simulink model "New_2"  (R2020a)
settings: Solver=VariableStepAuto  StartTime=0.0  StopTime=0.3  MaxStep=1e-5  RelTol=1e-3  EnableMultiTasking=on
libraries: simulink x1
settings Model: SimulationMode=accelerator  Creator=OXAALJ  LastModifiedBy=galarm2
settings SolverCC: MaxOrder=2  MaxConsecutiveZCs=10  MaxConsecutiveMinStep=10  ZeroCrossControl=DisableAll
settings DataIOCC: LimitDataPoints=on  SaveFormat=Array  DSMLogging=off  ReturnWorkspaceOutputs=off
settings OptimizationCC: LifeSpan=inf
settings DebuggingCC: UnderspecifiedInitializationDetection=Classic  MergeDetectMultiDrivingBlocksExec=none  SolverPrmCheckMsg=warning  MultiTaskDSMMsg=warning  MultiTaskCondExecSysMsg=none  StateNameClashWarn=warning  SFUnexpectedBacktrackingDiag=warning  SFNoUnconditionalDefaultTransitionDiag=warning  SFExecutionAtInitializationDiag=none  ArithmeticOperatorsInVariantConditions=warning
settings HardwareCC: ProdBitPerPointer=32  ProdBitPerSizeT=32  ProdBitPerPtrDiffT=32  ProdLargestAtomicFloat=None  ProdIntDivRoundTo=Undefined  ProdEndianess=Unspecified  ProdWordSize=32  ProdHWDeviceType=32-bit Generic
settings ModelReferenceCC: PropagateSignalLabelsOutOfModel=off
settings SFSimCC: SimUseLocalCustomCode=off  CustomCodeUndefinedFunction=UseInterfaceOnly
settings RTWCC: RTWUseLocalCustomCode=off
settings CodeAppCC: StateflowObjectComments=on
settings GRTTargetCC: TargetLangStandard=C89/C90 (ANSI)
settings ConfigComp: CovMetricSettings=dw  CovHtmlReporting=on  CovSaveCumulativeToWorkspaceVar=on  CovSaveSingleToWorkspaceVar=on  CovExternalEMLEnable=off  CovSFcnEnable=off

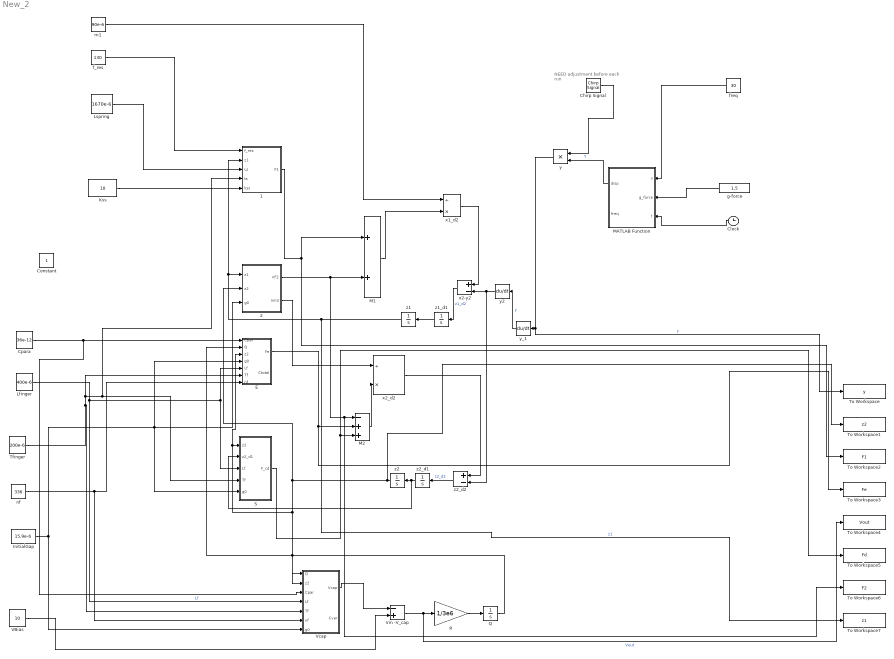
== system New_2 ==
  note: NEED
      | adjustment
      | before each
      | run
  " M1" : Sum  RndMeth=Nearest
  1 : MATLAB Function  TreatAsAtomicUnit=on
  2 : MATLAB Function  TreatAsAtomicUnit=on
  Chirp Signal : simulink/Sources/Chirp Signal  f1=30  T=0.3  f2=30
  Clock : Clock
  Cpara : Constant  Value=36e-12  VectorParams1D=off
  E : MATLAB Function  TreatAsAtomicUnit=on
  InitialGap : Constant  Value=15.9e-6
  Kss : Constant  Value=10
  Lfinger : Constant  Value=400e-6
  Lspring : Constant  Value=1670e-6
  M2 : Sum  Inputs=-++  RndMeth=Nearest
  MATLAB Function : MATLAB Function  TreatAsAtomicUnit=on
  Q : Integrator
  R : Gain  Gain=1/3e6
  S : MATLAB Function  TreatAsAtomicUnit=on
  Tfinger : Constant  Value=200e-6
  To Workspace : ToWorkspace  VariableName=y  SampleTime=-1
      settings: Save2DSignal=2-D array (concatenate along first dimension)
  To Workspace1 : ToWorkspace  VariableName=z2  SampleTime=-1
      settings: Save2DSignal=2-D array (concatenate along first dimension)
  To Workspace2 : ToWorkspace  VariableName=F1  SampleTime=-1
      settings: Save2DSignal=2-D array (concatenate along first dimension)
  To Workspace3 : ToWorkspace  VariableName=Fe  SampleTime=-1
      settings: Save2DSignal=2-D array (concatenate along first dimension)
  To Workspace4 : ToWorkspace  VariableName=Vout  SampleTime=-1
      settings: Save2DSignal=2-D array (concatenate along first dimension)
  To Workspace5 : ToWorkspace  VariableName=Fd  SampleTime=-1
      settings: Save2DSignal=2-D array (concatenate along first dimension)
  To Workspace6 : ToWorkspace  VariableName=F2  SampleTime=-1
      settings: Save2DSignal=2-D array (concatenate along first dimension)
  To Workspace7 : ToWorkspace  VariableName=z1  SampleTime=-1
      settings: Save2DSignal=2-D array (concatenate along first dimension)
  VBias : Constant  Value=10
  Vcap : MATLAB Function  TreatAsAtomicUnit=on
  Vin -V_cap : Sum  Inputs=-+  RndMeth=Nearest
  f_res : Constant  Value=130
  freq : Constant  Value=30
  g-force : Constant  Value=1.5
  m1 : Constant  Value=90e-6
  nf : Constant  Value=336
  x1_d2 : Product  Inputs=/*
  x2-y2 : Sum  Inputs=+-  RndMeth=Nearest
  x2_d2 : Product  Inputs=/*
  y : Product
  y2 : Derivative
  y_1 : Derivative
  z1 : Integrator
  z1_d1 : Integrator
  z2 : Integrator
  z2_d1 : Integrator
  z2_d2 : Sum  Inputs=+-  RndMeth=Nearest
  Constant : Constant  IOType=siggen
  wires:
  E/1(Fe) -> To Workspace3/1, M2/2
  1/1(F1) -> To Workspace2/1, " M1"/1
  S/1(F_cd) -> To Workspace5/1, M2/3
  f_res/1 -> 1/1(f_res)
  m1/1 -> x1_d2/1
  Clock/1 -> MATLAB Function/3(t)
  g-force/1 -> MATLAB Function/2(g_force)
  freq/1 -> MATLAB Function/1(f)
  MATLAB Function/1(disp) -> y/2  "Y"
  y/1 -> To Workspace/1, y_1/1  "y"
  InitialGap/1 -> E/4(g0), S/5(g0), 2/3(g0), Vcap/7(g0)
  VBias/1 -> Vin -V_cap/2
  Vin -V_cap/1 -> To Workspace4/1, R/1  "Vout"
  R/1 -> Q/1
  Q/1 -> E/2(Q), Vcap/1(Q)
  Vcap/1(Vcap) -> Vin -V_cap/1
  Lfinger/1 -> Vcap/4(Lf), E/5(Lf), S/3(Lf)  "Lf"
  Cpara/1 -> Vcap/3(Cpar), E/1(Cpar)
  Chirp Signal/1 -> y/1
  nf/1 -> Vcap/6(nf), E/7(nf)
  Lspring/1 -> 1/3(Ls)
  Tfinger/1 -> E/6(Tf), 1/4(ts), S/4(Tf), Vcap/5(Tf)
  Kss/1 -> 1/5(kss)
  2/1(nF2) -> To Workspace6/1, M2/1, " M1"/2
  " M1"/1 -> x1_d2/2
  y_1/1 -> y2/1  "y"
  x1_d2/1 -> x2-y2/1
  y2/1 -> z2_d2/2, x2-y2/2
  x2-y2/1 -> z1_d1/1  "z1_d2"
  z1_d1/1 -> z1/1
  z1/1 -> To Workspace7/1, 1/2(z1), 2/1(z1)  "z1"
  x2_d2/1 -> z2_d2/1
  z2_d2/1 -> z2_d1/1  "z2_d2"
  z2_d1/1 -> S/2(z2_d1), z2/1
  z2/1 -> To Workspace1/1, Vcap/2(z2), S/1(z2), E/3(z2), 2/2(z2)
  2/2(nm2) -> x2_d2/1
  M2/1 -> x2_d2/2

== matlab function New_2/E ==
  data: Cpar input; Q input; Fe output; z2 input; g0 input; Ctotal output; Lf input; Tf input; nf input
function [Fe,Ctotal] = fcn(Cpar,Q,z2,g0,Lf,Tf,nf)
% This function is to calculate the Fe (electrostatic force on m2)


%%%% slanted electrodes (BASSET 2014)
a = 3.5/200;    %aspect ratio
%C = ((eps0.*nf.*Lf)./(4.*a)).*log( ((g+2.*Wf.*a).^2 - z2.^2)./ (g.^2 - z2.^2));
% Cfit = (4.58916e18)*z2^6 - (6.34823e10)*z2^5 - (8.01379e8)*z2^4 + ...
%     (1.06902e1)*z2^3 + (8.85118e-2)*z2^2 + (3.66175e-11)*z2 + 1.50912e-11; % from excel
%Ctotal = Cfit + Cpar;
%==========================================================================
% Accounting for Parylene

eps0 = 8.85e-12;                                %permitivity of free space 
er   = 3.15;                                    %relative dielectric (Parylene C)
t    = 200e-9;                                  % thickness of parylene
g_p  = g0 - 2*t;                                % Minimum air gap
Ctot = 0;                                       % this gets reassigned in the if statements
z2lin = 1.54e-5;                              % z2 value at which linear approx starts
dcdz2 = 0.0605;                                % Slope of linear approx
c0 = 1.1855e-10;                                % Capacitance value at z2lin

if g_p > abs(z2)    %separate motion
    z2 = z2 * 2;
    C_L = ((eps0.*Lf)./(2.*a)).*( log( (g_p + z2 + 2.*a.*Tf)./(g_p + z2) ) );
    C_Leff = 1./( (2./(er.*eps0.*Lf.*Tf./t)) + 1./C_L);
    
    C_R = ((eps0.*Lf)./(2.*a)).*( log( (g_p - z2 + 2.*a.*Tf)./(g_p - z2) ) );
    C_Reff = 1 ./ ( (2./(er.*eps0.*Lf.*Tf./t)) + 1./C_R);

    Ctot = (C_Leff + C_Reff).*(nf./2);    
end

if -z2lin > z2      % Impacting with Left Hand side
    Ctot = c0 + dcdz2.*(-g_p - z2); 
end 

if z2 > z2lin      % impacting with RHS
    Ctot = c0 + dcdz2.*(z2 - g_p);
end

Ctotal = Ctot + Cpar;
% z2max = 15.5e-6;     %maximum displaccement for capacitance calc
% Cmax = (4.58916e18)*z2max^6 - (6.34823e10)*z2max^5 - (8.01379e8)*z2max^4 + ...
%     (1.06902e1)*z2max^3 + (8.85118e-2)*z2max^2 + (3.66175e-11)*z2max...
%     + 1.50912e-11;      %capacitance at z2max
% C = min(Cmax,Cfit);     % Use Cmax if z2>z2max


% dC is divided by four here because nf is total electrodes, not number of
% electrode pairs
dC = ((eps0.*nf.*Lf)./(4.*a))*( ((2*z2)/(g0^2 - z2^2)) - ((2*z2)/((g0+2*Tf*a)^2 - z2^2) ));

% dC = ((eps0.*nf.*Lf)./(1*a))*( ((2*z2)/(g0^2 - z2^2)) - ((2*z2)/((g0+2*Tf*a)^2 - z2^2) ));  % Nf IS the number of electrodes

Fe = -1*((Q^2)/(2*Ctotal^2))*dC;


end

== matlab function New_2/S ==
  data: z2 input; F_cd output; z2_d1 input; Lf input; Tf input; g0 input
function F_cd  = SQFD(z2,z2_d1,Lf,Tf,g0)
% This block supports an embeddable subset of the MATLAB language.
% See the help menu for details. 


mu = 1.846e-5;      %dynamic viscosity of air

%--------------------------------------------------------------------------
%Simple, low amplitude SQFD
% cd = nf*mu*Lf*Wf^3.*(1./(g-z).^3 + 1./(g+z).^3);
% A   = 14.4e-6;      %Soft Stopper Nominal Gap (meters)
% 
t    = 200e-9;                                  % thickness of parylene
g_p  = g0 - 2*t;                                % Minimum air gap


if  abs (z2) < g_p    %the separate motion
    z2 = 2*z2;
    z2_d1 = 2*z2_d1;
end   
% 
% b_eff   =   1.3;                                      % boarder effect coefficient
% epsr    =   3.15;                                     % relative dielectric
% 
% 
% tf_r    =   Tf + b_eff * ( g_p - z2 );
% tf_l    =   Tf + b_eff * ( g_p + z2 );
% lf_r    =   Lf + b_eff * ( g_p - z2 );
% lf_l    =   Lf + b_eff * ( g_p + z2 );
% 
% cdr     =   nf * mu * lf_r * tf_r^3 * ( g_p - z2  ) ^(-3) ;
% cdl     =   nf * mu * lf_l * tf_l^3 * ( g_p + z2  ) ^(-3) ;
% 
% F_cd      =   - 1*( cdr + cdl ) * z2_d1 ; 


%-----------The classic squeeze film damping equation------------%
% 
% tp        =   200e-9;                                     % the thickness of paralyene
% Cd        =   20e-20;  
% epsr      =   3.15;                                       % relative dielectric
% 
% F_cd        =   -Cd * z2_d1* (( g_p  - z2 + 2*tp/epsr) ^(-3) + ( g_p  + z2 + 2*tp/epsr) ^(-3));

%% Andy Moy damping original
% mu    =   1.983e-5;                                   %Air viscocity dynamic (kg/m*s)
% rho   =   1.204;                                      %Air density    (kg/m3)                    
% a     =   3.5*2/200;                                  %Tilt angle difference, tan(a)- tan(b)
% 
% 
% t    = 200e-9;                                  % thickness of parylene
% g_p  = g0 - 2*t;                                % Minimum air gap
% % Left-hand side
% 
% ho_l  =  g_p + z2;                                    %Left-hand side ho
% hl_l  =  ho_l + a*Tf;                                %Left-hand side hl
% 
% C1_l  =  -ho_l*Tf/(ho_l + 2*a)* z2_d1;               %The c1 parameter, left
% C2_l  =  12*mu*a^-2/(2*ho_l + a*Tf) * z2_d1;         %The c1 parameter, left
% 
% 
% F_l   =  Lf * (Tf * C2_l - 6*mu*Tf/a/ho_l/hl_l*C1_l + 6*mu*Tf*a^-4/hl_l*z2_d1+ 12*mu*a^-3 * z2_d1 * (log(ho_l./hl_l)) ); 
% % F_l   =  Lf * (Tf * C2_l - 6*mu*Tf/a/ho_l/hl_l*C1_l + 6*mu*Tf*a^-4/hl_l*z2_d1+ 12*mu*a^-3 * z2_d1 * (log(16/22)) ); 
% % Right-hand side                   
% 
% ho_r  =  g_p - z2;                                    %Left-hand side ho
% hl_r  =  ho_r + a*Tf;                                %Left-hand side hl
% 
% C1_r  =  -ho_r*Tf/(ho_r + 2*a)* z2_d1;                 %The c1 parameter, right
% C2_r  =  12*mu*a^-2/(2*ho_r + a*Tf) * z2_d1;         %The c1 parameter, right
% 
% 
% F_r   =  Lf * (Tf * C2_r - 6*mu*Tf/a/ho_r/hl_r*C1_r + 6*mu*Tf*a^-4/hl_r*z2_d1 + 12*mu*a^-3 * z2_d1 * (log(ho_r./hl_r) )) ; 
% % F_r   =  Lf * (Tf * C2_r - 6*mu*Tf/a/ho_r/hl_r*C1_r + 6*mu*Tf*a^-4/hl_r*z2_d1 + 12*mu*a^-3 * z2_d1 * (log(16/22) )) ; 
% F_cd  =  -100000*(F_l  + F_r)*nf;


%% Andy Moy damping Tf Lf
mu    =   1.983e-5;                                   %Air viscocity dynamic (kg/m*s)
rho   =   1.204;                                      %Air density    (kg/m3)                    
a     =   3.5*2/200;                                  %Tilt angle difference, tan(a)- tan(b)


t    = 200e-9;                                  % thickness of parylene
g_p  = g0 - 2*t;                                % Minimum air gap
% Left-hand side

ho_l  =  g_p + z2;                                    %Left-hand side ho
hl_l  =  ho_l + a*Lf;                                %Left-hand side hl

C1_l  =  -ho_l*Lf/(ho_l + 2*a)* z2_d1;               %The c1 parameter, left
C2_l  =  12*mu*a^-2/(2*ho_l + a*Lf) * z2_d1;         %The c1 parameter, left


F_l   =  Tf * (Lf * C2_l - 6*mu*Lf/a/ho_l/hl_l*C1_l + 6*mu*Lf*a^-4/hl_l*z2_d1+ 12*mu*a^-3 * z2_d1 * (log(ho_l./hl_l)) )*0.336; 
% F_l   =  Lf * (Tf * C2_l - 6*mu*Tf/a/ho_l/hl_l*C1_l + 6*mu*Tf*a^-4/hl_l*z2_d1+ 12*mu*a^-3 * z2_d1 * (log(16/22)) ); 
% Right-hand side                   

ho_r  =  g_p - z2;                                    %Left-hand side ho
hl_r  =  ho_r + a*Lf;                                %Left-hand side hl

C1_r  =  -ho_r*Lf/(ho_r + 2*a)* z2_d1;                 %The c1 parameter, right
C2_r  =  12*mu*a^-2/(2*ho_r + a*Lf) * z2_d1;         %The c1 parameter, right


F_r   =  Tf * (Lf * C2_r - 6*mu*Lf/a/ho_r/hl_r*C1_r + 6*mu*Lf*a^-4/hl_r*z2_d1 + 12*mu*a^-3 * z2_d1 * (log(ho_r./hl_r) ))*0.336 ; 
% F_r   =  Lf * (Tf * C2_r - 6*mu*Tf/a/ho_r/hl_r*C1_r + 6*mu*Tf*a^-4/hl_r*z2_d1 + 12*mu*a^-3 * z2_d1 * (log(16/22) )) ; 
F_cd  =  -(F_l  + F_r);

end

== matlab function New_2/2 ==
  data: z1 input; z2 input; nF2 output; g0 input; nm2 output
function [nF2, nm2] = fcn(z1, z2, g0)

%% Jinglun Li, lij31@rpi.edu/06/14/2019
% This is to calculate the F2 on m1 and m2, which is:

% Inputs:

% The displacement (z1)
% The displacement (z2)
% The effective spring constant k2 

% Output:
%  F2 = -k2 * (z1 - z2)

%% k2
t    = 200e-9;                                  % thickness of parylene
g_p  = g0 - 2*t;                                % Minimum air gap



 if       abs (z2) < g_p 
          nm2      =    0.1e-8;                                   % Cantilever's mass
          nk2      =    3000;                                     % Spring constant from movable electrodes
          nF2       =   - nk2*(z1 - z2);                           % From the second spring       

 
 
 else

          nm2      =    0.2e-8;                                   % Cantilever's mass
          nk2      =    3000;
          nF2       =   - nk2*(z1 - z2)+ nk2*z2;                    % From the second spring     
 end

%% Force calculation

end

== matlab function New_2/MATLAB Function ==
  data: f input; disp output; g_force input; t input; freq output
function [disp,freq] = fcn(f,g_force,t)
%#codegen
% accel = g_force*9.81;

ramp = 200e-3;

if t < ramp
   freq = f;
   disp = (t/ramp)* (g_force/(4.0243*freq^2));          %const = (2*pi())^2/9.81
%         vel = (t/ramp)*(g_force*9.81)/(2*pi*freq);
else
    freq = f;
    disp = g_force/(4.0243*freq^2);          %const = (2*pi())^2/9.81
%   vel = (g_force*9.81)/(2*pi*freq);
%   disp = g/(4.0243*((fhigh-flow)/2)^2); 

%   freq = (0.5) * (fhigh+flow);
%   disp = g/(4.0243*freq^2);          %const = (2*pi())^2/9.81
end

% freq = (t/sweep_time)*(fhigh-flow) + flow;
% freq = (0.5) * (fhigh+flow);
% disp = g/(4.0243*freq^2);          %const = (2*pi())^2/9.81
% disp = g/(4.0243*((fhigh-flow)/2)^2); 

% coder.extrinsic('chirp');
% y = chirp(t,flow,sweep_time,fhigh,'linear',0);
% y_dot = chirp(t,flow,sweep_time,fhigh,'linear',90);
% y_dot_dot = chirp(t,flow,sweep_time,fhigh,'linear',180);

end

== matlab function New_2/1 ==
  data: f_res input; z1 input; F1 output; Ls input; ts input; kss input
function F1 = fcn(f_res,z1, Ls, ts, kss)

%% Jinglun Li, lij31@rpi.edu/06/14/2019
% This is to calculate the F1 on m1, which is:

% Inputs:
% The measuerd resonant frequency of m1
% The spring length of suspension spring
% The device thickness
% The spring constant of the softspring attache to the anchor
% The displacement (z11)


% Output:
%  F1 = Fsp +  Fss
%  Fsp - from the suspension spring
%  Fss - from the 


%% The device parameters, format should be constant ( all in SI unit)
m1     =     90e-6;
E      =     180e9;                                   % The Young's mudulous 
ws     =    10e-6;                                   % spring width (m)


% Parameters from back calculation


% 
A  = 14.4e-6;      %Soft Stopper Nominal Gap (meters)
g0 = 15.91e-6;      % Nominal Gap (m)
B  = 15.5e-6;      % Parylene stopper gap (m)... B = g0 - 2*200nm


% % Back Calculate effective spring beam width
omega0   =    f_res*2*pi;                             %The measured fresonant angular frequency                       
k1       =    (omega0)^2*m1;                          %Linear spring constant k1 (N/m)
wseff    = (((Ls^3)*k1)/(2*E*ts))^(1/3);         %effective spring beam width (m)
k3_singu = (18/25)*(k1/2)*(1/(wseff^2));         %cubic spring constant of a single spring,  k3 (N/m)
k3       = k3_singu/8;                           %k3 of all the connected suspension springs
% 

% k1      =    2*E *ts*(ws^3)/(Ls^3);                       % Spring constant from supporting beams
% k3      =    1/2*(18/25)*E * ts*ws/(Ls^3);


%% Force calculation
% Fsp      =  -k1.*z1 - k3.*z1.^3;                 %Spring force from the suspension spring (N)
Fsp      =  -k1.*z1 - k3*1*(z1^3);                 %Spring force from the suspension spring (N)

%  Fss: to execute the piece-wise function

% To execute the piece-wise function
    if     abs (z1) < A
         Fss = 0;                                %No stoppers 
    else
         Fss = - kss*(z1-A)*sign(z1);          %Soft stopper
    end

F1       =   Fsp  +  Fss;                        %The spring force F1       


end

== matlab function New_2/Vcap ==
  data: Q input; z2 input; Vcap output; Cpar input; Cvar output; Lf input; Tf input; nf input; g0 input
function [Vcap,Cvar]  = fcn(Q, z2, Cpar, Lf,Tf,nf, g0)
%#codegen
eps0 = 8.85e-12;


% %%%% slanted electrodes (BASSET 2014)
a = 3.5/200;
%C = ((eps0.*nf.*Lf)./(4.*a)).*log( ((g+2.*Wf.*a).^2 - z.^2)./ (g.^2 - z.^2));
% Cfit = (4.58916e18)*z^6 - (6.34823e10)*z^5 - (8.01379e8)*z^4 + ...
%     (1.06902e1)*z^3 + (8.85118e-2)*z^2 + (3.66175e-11)*z + 1.50912e-11; % from excel
% Cvar = Cfit + Cpar;

% zmax = 15.5e-6;     %maximum displaccement for capacitance calc
% Cmax = (4.58916e18)*zmax^6 - (6.34823e10)*zmax^5 - (8.01379e8)*zmax^4 + ...
%     (1.06902e1)*zmax^3 + (8.85118e-2)*zmax^2 + (3.66175e-11)*zmax...
%     + 1.50912e-11;      %capacitance at zmax
% C = min(Cmax,Cfit);     % Use Cmax if z>zmax


%==========================================================================
% Accounting for Parylene
er = 3.15;          % relative dielectric
t = 200e-9;         % thickness of parylene

g_p  = g0 - 2*t;                                % Minimum air gap
Ctot = 0;           % this gets reassigned in the if statements
Zlin = 1.54e-5;   % z value at which linear approx starts
dcdz = 0.0605;     % Slope of linear approx
c0 = 1.1855e-10;    % Capacitance value at Zlin

if g_p > abs(z2)
    z2 = z2 * 2;
    
    C_L = ((eps0.*Lf)./(2.*a)).*( log( (g_p + z2 + 2.*a.*Tf)./(g_p + z2) ) );
    C_Leff = 1./( (2./(er.*eps0.*Lf.*Tf./t)) + 1./C_L);
    
    C_R = ((eps0.*Lf)./(2.*a)).*( log( (g_p - z2 + 2.*a.*Tf)./(g_p - z2) ) );
    C_Reff = 1 ./ ( (2./(er.*eps0.*Lf.*Tf./t)) + 1./C_R);

    Ctot = (C_Leff + C_Reff).*(nf);    
end

if -Zlin > z2      % Impacting with Left Hand side
    Ctot = c0 + dcdz.*(-g_p - z2); 
end 

if z2 > Zlin      % impacting with RHS
    Ctot = c0 + dcdz.*(z2 - g_p);
end


Cvar = Ctot + Cpar;
%==========================================================================

Vcap = Q/Cvar;
end
